simulink model "control"  (R2014a)
settings: Solver=ode1  StartTime=0.0  StopTime=inf  FixedStep=Ts  RelTol=1e-3
InitFcn:
  | control_initfcn
StopFcn:
  | control_stopfcn
undefined symbols (not defined in the file): armSide, cobot4a, dataLoggerStartTime, dataLoggerStopTime, forgettingFactor, g, initializationTime, initOrientationLeftArmTwo, initOrientationRightArmTwo, initPositionLeftArm, initPositionRightArm, MANIPULATION_CMD_CONFIGURATION, MANIPULATION_CMD_CONFIGURATION_VELOCITY, matterhorn, maxTime, minTime, rampTime, rotationAmplitude, rotationFrequency, rotationPhaseShift, timeForMovement, translationAmplitude, translationFrequency, translationPhaseShift, Ts, vxMax, vyMax, vzMax, wxMax, wyMax, wzMax, xMax, xMin, yMax, yMin, zMax, zMin
libraries: rtai_devices x42, dsparch4 x39, sfbc_lib x6, simulink x2, rtai_utilities x2
(part 2 of 2)

== system control/Measurement/Data Acquisition/QualisysTracker ==
  SFBcomm receiver : sfbc_lib/SFBcomm receiver  localPort=33000  streamID=1  remoteSettings=127.0.0.1:34000  portNames=A  portWidths=32  outputLatency=off  outputIdleTime=off  connectTimeout=50  sampleTime=-1
  Selector : Selector  InputPortWidth=32  Indices=1:8
  Selector1 : Selector  InputPortWidth=32  Indices=9:16
  Selector2 : Selector  InputPortWidth=32  Indices=17:24
  Selector3 : Selector  InputPortWidth=32  Indices=25:32
  EndEffektorFrame : Outport
  RobotFrame : Outport  Port=2
  HandleLeft : Outport  Port=3
  HandleRight : Outport  Port=4
  wires:
  SFBcomm receiver/1 -> Selector/1, Selector3/1, Selector2/1, Selector1/1
  Selector3/1 -> HandleRight/1
  Selector2/1 -> HandleLeft/1
  Selector1/1 -> EndEffektorFrame/1
  Selector/1 -> RobotFrame/1

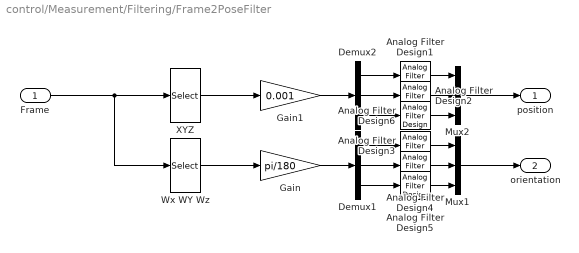
== system control/Measurement/Filtering/Frame2PoseFilter ==
  Frame : Inport
  Analog Filter Design{1..4} (4 alike) : dsparch4/Analog Filter Design  method=Butterworth  filttype=Lowpass  N=2  Wlo=cutOffFrequ  Whi=80  Rp=2  Rs=40
  Analog Filter Design5 : dsparch4/Analog Filter Design  method=Butterworth  filttype=Lowpass  N=3  Wlo=cutOffFrequ  Whi=80  Rp=2  Rs=40
  Analog Filter Design6 : dsparch4/Analog Filter Design  method=Butterworth  filttype=Lowpass  N=3  Wlo=cutOffFrequ  Whi=80  Rp=2  Rs=40
  Demux1 : Demux  Outputs=3
  Demux2 : Demux  Outputs=3
  Gain : Gain  Gain=pi/180
  Gain1 : Gain  Gain=0.001
  Mux1 : Mux  Inputs=3
  Mux2 : Mux  Inputs=3
  Wx WY Wz : Selector  InputPortWidth=8  Indices=[6:8]
  XYZ : Selector  InputPortWidth=8  Indices=[3:5]
  position : Outport
  orientation : Outport  Port=2
  wires:
  Wx WY Wz/1 -> Gain/1
  Frame/1 -> Wx WY Wz/1, XYZ/1
  XYZ/1 -> Gain1/1
  Demux1/1 -> Analog Filter Design3/1
  Demux1/2 -> Analog Filter Design4/1
  Demux1/3 -> Analog Filter Design5/1
  Analog Filter Design5/1 -> Mux1/3
  Analog Filter Design3/1 -> Mux1/1
  Analog Filter Design4/1 -> Mux1/2
  Demux2/1 -> Analog Filter Design1/1
  Demux2/2 -> Analog Filter Design2/1
  Demux2/3 -> Analog Filter Design6/1
  Gain/1 -> Demux1/1
  Mux1/1 -> orientation/1
  Gain1/1 -> Demux2/1
  Analog Filter Design6/1 -> Mux2/3
  Analog Filter Design1/1 -> Mux2/1
  Analog Filter Design2/1 -> Mux2/2
  Mux2/1 -> position/1

== system control/Measurement/Filtering/Frame2PoseFilter1 ==
  Frame : Inport
  Analog Filter Design3 : dsparch4/Analog Filter Design  method=Butterworth  filttype=Lowpass  N=2  Wlo=cutOffFrequ  Whi=80  Rp=2  Rs=40
  Analog Filter Design4 : dsparch4/Analog Filter Design  method=Butterworth  filttype=Lowpass  N=2  Wlo=cutOffFrequ  Whi=80  Rp=2  Rs=40
  Analog Filter Design5 : dsparch4/Analog Filter Design  method=Butterworth  filttype=Lowpass  N=3  Wlo=cutOffFrequ  Whi=80  Rp=2  Rs=40
  Demux1 : Demux  Outputs=3
  Gain : Gain  Gain=pi/180
  Mux1 : Mux  Inputs=3
  Wx WY Wz : Selector  InputPortWidth=8  Indices=[6:8]
  orientation : Outport
  wires:
  Wx WY Wz/1 -> Gain/1
  Frame/1 -> Wx WY Wz/1
  Demux1/1 -> Analog Filter Design3/1
  Demux1/2 -> Analog Filter Design4/1
  Demux1/3 -> Analog Filter Design5/1
  Analog Filter Design5/1 -> Mux1/3
  Analog Filter Design3/1 -> Mux1/1
  Analog Filter Design4/1 -> Mux1/2
  Gain/1 -> Demux1/1
  Mux1/1 -> orientation/1

== system control/Measurement/Filtering/Frame2PoseFilter2 ==
  Frame : Inport
  Analog Filter Design{1..4} (4 alike) : dsparch4/Analog Filter Design  method=Butterworth  filttype=Lowpass  N=2  Wlo=cutOffFrequ  Whi=80  Rp=2  Rs=40
  Analog Filter Design5 : dsparch4/Analog Filter Design  method=Butterworth  filttype=Lowpass  N=3  Wlo=cutOffFrequ  Whi=80  Rp=2  Rs=40
  Analog Filter Design6 : dsparch4/Analog Filter Design  method=Butterworth  filttype=Lowpass  N=3  Wlo=cutOffFrequ  Whi=80  Rp=2  Rs=40
  Demux1 : Demux  Outputs=3
  Demux2 : Demux  Outputs=3
  Gain : Gain  Gain=pi/180
  Gain1 : Gain  Gain=0.001
  Mux1 : Mux  Inputs=3
  Mux2 : Mux  Inputs=3
  Wx WY Wz : Selector  InputPortWidth=8  Indices=[6:8]
  XYZ : Selector  InputPortWidth=8  Indices=[3:5]
  position : Outport
  orientation : Outport  Port=2
  wires:
  Wx WY Wz/1 -> Gain/1
  Frame/1 -> Wx WY Wz/1, XYZ/1
  XYZ/1 -> Gain1/1
  Demux1/1 -> Analog Filter Design3/1
  Demux1/2 -> Analog Filter Design4/1
  Demux1/3 -> Analog Filter Design5/1
  Analog Filter Design5/1 -> Mux1/3
  Analog Filter Design3/1 -> Mux1/1
  Analog Filter Design4/1 -> Mux1/2
  Demux2/1 -> Analog Filter Design1/1
  Demux2/2 -> Analog Filter Design2/1
  Demux2/3 -> Analog Filter Design6/1
  Gain/1 -> Demux1/1
  Mux1/1 -> orientation/1
  Gain1/1 -> Demux2/1
  Analog Filter Design6/1 -> Mux2/3
  Analog Filter Design1/1 -> Mux2/1
  Analog Filter Design2/1 -> Mux2/2
  Mux2/1 -> position/1

== system control/Measurement/Filtering/Frame2PoseFilter3 ==
  Frame : Inport
  Analog Filter Design{1..4} (4 alike) : dsparch4/Analog Filter Design  method=Butterworth  filttype=Lowpass  N=2  Wlo=cutOffFrequ  Whi=80  Rp=2  Rs=40
  Analog Filter Design5 : dsparch4/Analog Filter Design  method=Butterworth  filttype=Lowpass  N=3  Wlo=cutOffFrequ  Whi=80  Rp=2  Rs=40
  Analog Filter Design6 : dsparch4/Analog Filter Design  method=Butterworth  filttype=Lowpass  N=3  Wlo=cutOffFrequ  Whi=80  Rp=2  Rs=40
  Demux1 : Demux  Outputs=3
  Demux2 : Demux  Outputs=3
  Gain : Gain  Gain=pi/180
  Gain1 : Gain  Gain=0.001
  Mux1 : Mux  Inputs=3
  Mux2 : Mux  Inputs=3
  Wx WY Wz : Selector  InputPortWidth=8  Indices=[6:8]
  XYZ : Selector  InputPortWidth=8  Indices=[3:5]
  position : Outport
  orientation : Outport  Port=2
  wires:
  Wx WY Wz/1 -> Gain/1
  Frame/1 -> Wx WY Wz/1, XYZ/1
  XYZ/1 -> Gain1/1
  Demux1/1 -> Analog Filter Design3/1
  Demux1/2 -> Analog Filter Design4/1
  Demux1/3 -> Analog Filter Design5/1
  Analog Filter Design5/1 -> Mux1/3
  Analog Filter Design3/1 -> Mux1/1
  Analog Filter Design4/1 -> Mux1/2
  Demux2/1 -> Analog Filter Design1/1
  Demux2/2 -> Analog Filter Design2/1
  Demux2/3 -> Analog Filter Design6/1
  Gain/1 -> Demux1/1
  Mux1/1 -> orientation/1
  Gain1/1 -> Demux2/1
  Analog Filter Design6/1 -> Mux2/3
  Analog Filter Design1/1 -> Mux2/1
  Analog Filter Design2/1 -> Mux2/2
  Mux2/1 -> position/1

== system control/Measurement/Filtering/signalFilt ==
  sigIn : Inport
  Analog Filter Design1 : dsparch4/Analog Filter Design  method=Butterworth  filttype=Lowpass  N=2  Wlo=cutOffFrequ  Whi=80  Rp=2  Rs=40
  Analog Filter Design2 : dsparch4/Analog Filter Design  method=Butterworth  filttype=Lowpass  N=2  Wlo=cutOffFrequ  Whi=80  Rp=2  Rs=40
  Analog Filter Design6 : dsparch4/Analog Filter Design  method=Butterworth  filttype=Lowpass  N=3  Wlo=cutOffFrequ  Whi=80  Rp=2  Rs=40
  Demux2 : Demux  Outputs=3
  Mux2 : Mux  Inputs=3
  sigOut : Outport
  wires:
  Demux2/1 -> Analog Filter Design1/1
  Demux2/2 -> Analog Filter Design2/1
  Demux2/3 -> Analog Filter Design6/1
  Analog Filter Design6/1 -> Mux2/3
  Analog Filter Design1/1 -> Mux2/1
  Analog Filter Design2/1 -> Mux2/2
  Mux2/1 -> sigOut/1
  sigIn/1 -> Demux2/1

== system control/Measurement/Filtering/signalFilt1 ==
  sigIn : Inport
  Analog Filter Design1 : dsparch4/Analog Filter Design  method=Butterworth  filttype=Lowpass  N=2  Wlo=cutOffFrequ  Whi=80  Rp=2  Rs=40
  Analog Filter Design2 : dsparch4/Analog Filter Design  method=Butterworth  filttype=Lowpass  N=2  Wlo=cutOffFrequ  Whi=80  Rp=2  Rs=40
  Analog Filter Design6 : dsparch4/Analog Filter Design  method=Butterworth  filttype=Lowpass  N=3  Wlo=cutOffFrequ  Whi=80  Rp=2  Rs=40
  Demux2 : Demux  Outputs=3
  Mux2 : Mux  Inputs=3
  sigOut : Outport
  wires:
  Demux2/1 -> Analog Filter Design1/1
  Demux2/2 -> Analog Filter Design2/1
  Demux2/3 -> Analog Filter Design6/1
  Analog Filter Design6/1 -> Mux2/3
  Analog Filter Design1/1 -> Mux2/1
  Analog Filter Design2/1 -> Mux2/2
  Mux2/1 -> sigOut/1
  sigIn/1 -> Demux2/1

== system control/Measurement/Filtering/signalFilt2 ==
  sigIn : Inport
  Analog Filter Design1 : dsparch4/Analog Filter Design  method=Butterworth  filttype=Lowpass  N=2  Wlo=cutOffFrequ  Whi=80  Rp=2  Rs=40
  Analog Filter Design2 : dsparch4/Analog Filter Design  method=Butterworth  filttype=Lowpass  N=2  Wlo=cutOffFrequ  Whi=80  Rp=2  Rs=40
  Analog Filter Design6 : dsparch4/Analog Filter Design  method=Butterworth  filttype=Lowpass  N=3  Wlo=cutOffFrequ  Whi=80  Rp=2  Rs=40
  Demux2 : Demux  Outputs=3
  Mux2 : Mux  Inputs=3
  sigOut : Outport
  wires:
  Demux2/1 -> Analog Filter Design1/1
  Demux2/2 -> Analog Filter Design2/1
  Demux2/3 -> Analog Filter Design6/1
  Analog Filter Design6/1 -> Mux2/3
  Analog Filter Design1/1 -> Mux2/1
  Analog Filter Design2/1 -> Mux2/2
  Mux2/1 -> sigOut/1
  sigIn/1 -> Demux2/1

== system control/Measurement/Filtering/signalFilt3 ==
  sigIn : Inport
  Analog Filter Design1 : dsparch4/Analog Filter Design  method=Butterworth  filttype=Lowpass  N=2  Wlo=cutOffFrequ  Whi=80  Rp=2  Rs=40
  Analog Filter Design2 : dsparch4/Analog Filter Design  method=Butterworth  filttype=Lowpass  N=2  Wlo=cutOffFrequ  Whi=80  Rp=2  Rs=40
  Analog Filter Design6 : dsparch4/Analog Filter Design  method=Butterworth  filttype=Lowpass  N=3  Wlo=cutOffFrequ  Whi=80  Rp=2  Rs=40
  Demux2 : Demux  Outputs=3
  Mux2 : Mux  Inputs=3
  sigOut : Outport
  wires:
  Demux2/1 -> Analog Filter Design1/1
  Demux2/2 -> Analog Filter Design2/1
  Demux2/3 -> Analog Filter Design6/1
  Analog Filter Design6/1 -> Mux2/3
  Analog Filter Design1/1 -> Mux2/1
  Analog Filter Design2/1 -> Mux2/2
  Mux2/1 -> sigOut/1
  sigIn/1 -> Demux2/1

== system control/Measurement/Filtering/signalFilt4 ==
  sigIn : Inport
  Analog Filter Design1 : dsparch4/Analog Filter Design  method=Butterworth  filttype=Lowpass  N=2  Wlo=cutOffFrequ  Whi=80  Rp=2  Rs=40
  Analog Filter Design2 : dsparch4/Analog Filter Design  method=Butterworth  filttype=Lowpass  N=2  Wlo=cutOffFrequ  Whi=80  Rp=2  Rs=40
  Analog Filter Design6 : dsparch4/Analog Filter Design  method=Butterworth  filttype=Lowpass  N=3  Wlo=cutOffFrequ  Whi=80  Rp=2  Rs=40
  Demux2 : Demux  Outputs=3
  Mux2 : Mux  Inputs=3
  sigOut : Outport
  wires:
  Demux2/1 -> Analog Filter Design1/1
  Demux2/2 -> Analog Filter Design2/1
  Demux2/3 -> Analog Filter Design6/1
  Analog Filter Design6/1 -> Mux2/3
  Analog Filter Design1/1 -> Mux2/1
  Analog Filter Design2/1 -> Mux2/2
  Mux2/1 -> sigOut/1
  sigIn/1 -> Demux2/1

== system control/Measurement/Filtering/signalFilt5 ==
  sigIn : Inport
  Analog Filter Design1 : dsparch4/Analog Filter Design  method=Butterworth  filttype=Lowpass  N=2  Wlo=cutOffFrequ  Whi=80  Rp=2  Rs=40
  Analog Filter Design2 : dsparch4/Analog Filter Design  method=Butterworth  filttype=Lowpass  N=2  Wlo=cutOffFrequ  Whi=80  Rp=2  Rs=40
  Analog Filter Design6 : dsparch4/Analog Filter Design  method=Butterworth  filttype=Lowpass  N=3  Wlo=cutOffFrequ  Whi=80  Rp=2  Rs=40
  Demux2 : Demux  Outputs=3
  Mux2 : Mux  Inputs=3
  sigOut : Outport
  wires:
  Demux2/1 -> Analog Filter Design1/1
  Demux2/2 -> Analog Filter Design2/1
  Demux2/3 -> Analog Filter Design6/1
  Analog Filter Design6/1 -> Mux2/3
  Analog Filter Design1/1 -> Mux2/1
  Analog Filter Design2/1 -> Mux2/2
  Mux2/1 -> sigOut/1
  sigIn/1 -> Demux2/1

== stateflow chart control/Master State Machine ==
  state INIT_POSE_CONTROL
    during: signalSelect = 1;
  state ESTIMATION_CONTROL
    during: signalSelect = 2;
  state MOVE_CONTROL
    during: signalSelect = 3;
  state INIT
    during: signalSelect = 4;
  state STOP
    during: signalSelect = 4;
  INIT -> INIT_POSE_CONTROL : [ACTIVATE_MANIPULATOR == 1]
  INIT_POSE_CONTROL -> ESTIMATION_CONTROL [order 2] : [ACTIVATE_ESTIMATION == 1 && after(initializationTime,sec)]
  ESTIMATION_CONTROL -> MOVE_CONTROL [order 2] : [ACTIVATE_MOVE == 1]
  (default) -> INIT
  INIT_POSE_CONTROL -> STOP [order 1] : [ACTIVATE_MANIPULATOR == 0]
  ESTIMATION_CONTROL -> STOP [order 1] : [ACTIVATE_MANIPULATOR == 0 || ACTIVATE_ESTIMATION == 0]
  MOVE_CONTROL -> STOP : [ACTIVATE_MANIPULATOR == 0]
  data: ACTIVATE_MANIPULATOR input; signalSelect output; ACTIVATE_ESTIMATION input; ACTIVATE_MOVE input; initializationTime input

== matlab function control/Actuator Interface/Guard ==
  data: u output; command input; velocityId input; positionId input
function u = fcn(command,velocityId,positionId)



streamId = command(1);

if((streamId == velocityId || streamId == positionId) && length(command) == 23)
    u = command;
else
	u = [velocityId;zeros(22,1)];
end

== matlab function control/Estimation Control/Parameter Estimation/Load Dynamics Estimation Three Grasping Points ==
  data: F1 input; thetaHat output; F2 input; F3 input; N1 input; N2 input; N3 input; omega input; domega input; ddp input; g input; r12 input; r13 input; forgettingFactor input; reinitialize input
function thetaHat = fcn(F1, F2, F3, N1, N2, N3, omega, domega, ddp, g, r12, r13, forgettingFactor,reinitialize)
    thetaHat = estimationThreeGraspingPoints(F1, F2, F3, N1, N2, N3, omega, domega, ddp, g, r12, r13, forgettingFactor, reinitialize);
end

== matlab function control/Measurement/Coordinate System Transformation/HandleLefttoWorld ==
  data: phi input; R output
function R = fcn(phi)
    R = createRotationMatrixLocalToGlobal(phi);
end

== matlab function control/Actuator Interface/IdSelector ==
  data: streamId input; u output; velocityId input; positionId input
function u = fcn(streamId,velocityId,positionId)

switch(streamId)
    case velocityId
        u = 1;
    case positionId
        u = 0;
    otherwise
        u = 1;
end

== matlab function control/Measurement/Coordinate System Transformation/RobottoWorld ==
  data: phi input; R output
function R = fcn(phi)
    R = createRotationMatrixLocalToGlobal(phi);
end

== matlab function control/Measurement/Offset Compensation/MATLAB Function ==
  data: trigger input; Force_Out output; Force input; Torque input; Torque_Out output; State output
function [Force_Out, Torque_Out, State] = fcn(trigger,Force,Torque)
[Force_Out, Torque_Out, State] = offsetCompensation(trigger,Force,Torque);
end

== matlab function control/Estimation Control/Trajectory Generator ==
  data: active input; u output; time input; translationAmplitude input; rotationAmplitude input; translationFrequency input; rotationFrequency input; translationPhaseShift input; rotationPhaseShift input; rampTime input
function u  = fcn(active, time, translationAmplitude, rotationAmplitude, translationFrequency, rotationFrequency, translationPhaseShift, rotationPhaseShift, rampTime)

persistent timeOffset activePrevious;

if(isempty(timeOffset))
    timeOffset = 0;
end

if(isempty(activePrevious))
    activePrevious = 0;
end

if (active == 1 && activePrevious == 0)
    timeOffset = time;
end

if (active == 1)
    timeWithoutOffset = time - timeOffset;
    amplitudes = [translationAmplitude; rotationAmplitude];
    frequencies = [translationFrequency; rotationFrequency];
    phaseShifts = [translationPhaseShift; rotationPhaseShift];
    u = amplitudes.*sin(frequencies.*timeWithoutOffset + phaseShifts);
    
    if (timeWithoutOffset < rampTime)
        u = u*timeWithoutOffset/rampTime;
    end
else
    u = zeros(6, 1);
end

activePrevious = active;

== matlab function control/Measurement/Coordinate System Transformation/EEFtoWorld ==
  data: phi input; R output
function R = fcn(phi)
    R = createRotationMatrixLocalToGlobal(phi);
end

== matlab function control/Measurement/Coordinate System Transformation/HandleRighttoWorld ==
  data: phi input; R output
function R = fcn(phi)
    R = createRotationMatrixLocalToGlobal(phi);
end

== matlab function control/Measurement/Offset Compensation1/MATLAB Function ==
  data: trigger input; Force_Out output; Force input; Torque input; Torque_Out output; State output
function [Force_Out, Torque_Out, State] = fcn(trigger,Force,Torque)
[Force_Out, Torque_Out, State] = offsetCompensation(trigger,Force,Torque);
end

== matlab function control/Measurement/Offset Compensation2/MATLAB Function ==
  data: trigger input; Force_Out output; Force input; Torque input; Torque_Out output; State output
function [Force_Out, Torque_Out, State] = fcn(trigger,Force,Torque)
[Force_Out, Torque_Out, State] = offsetCompensation(trigger,Force,Torque);
end

== matlab function control/MATLAB Function ==
  data: moto1 output size=[1, 4]; moto2 output size=[1, 4]; moto3 output size=[1, 4]; moto4 output size=[1, 4]
function [moto1, moto2, moto3, moto4 ] = processWarning
%#codegen

numVibes = 5;
defaultPeriod = 0.2;
defaultPhase = 0.0;
defaultDutyCycle = 0.25;

    
moto1 = [ defaultPeriod, defaultPhase, 1, numVibes ];
moto2 = [ defaultPeriod, defaultPhase, 1, numVibes ];
moto3 = [ defaultPeriod, defaultPhase, 1, numVibes ];
moto4 = [ defaultPeriod, defaultPhase, 1, numVibes ];
